simulink model "ControlSM_Tilt"  (R2013b)
settings: Solver=FixedStepDiscrete  StartTime=0.0  StopTime=10.0  FixedStep=0.001  RelTol=1e-3
undefined symbols (not defined in the file): B0, B13, B14, B3, C0, C9, DiscIntNeverNeededParam, P0, P13, P14, P16, P25, P3, Pin, Timer
libraries: MCHP_Blockset x13, simulink x1
settings Model: Creator=Residente  LastModifiedBy=Maestria01
settings OptimizationCC: InlineParams=on  InlineInvariantSignals=on  OptimizeModelRefInitCode=on  LifeSpan=1
settings HardwareCC: ProdBitPerInt=16  ProdBitPerPointer=16  ProdLargestAtomicInteger=Integer  ProdIntDivRoundTo=Zero  ProdEndianess=LittleEndian  ProdWordSize=16  ProdHWDeviceType=Generic->Custom
settings RTWCC: SystemTargetFile=MCHP_dsPIC_stf.tlc  TemplateMakefile=MCHP_dsPIC.tmf  Description=Microchip Embedded Target PIC24 dsPIC30 dsPIC33 (real-time)  ProcessScript=MCHP_dsPIC_stf_make_rtw_hook  CustomInclude=./Source  CustomSource=receive.c
settings CodeAppCC: IgnoreCustomStorageClasses=off
settings STFCustomTargetCC: TargetLibSuffix=_lib.a  IncludeMdlTerminateFcn=off  CombineOutputUpdateFcns=on  SuppressErrorStatus=on  ERTCustomFileBanners=on  SupportContinuousTime=off  MATLABClassNameForMDSCustomization=Simulink.SoftwareTarget.ERTCustomization  GRTInterface=off  SystemTargetFile=MCHP_dsPIC_stf.tlc
settings ERTTargetCC: TargetLibSuffix=_lib.a  CodeReplacementLibrary=ANSI_C  ParMdlRefBuildCompliant=off  CompOptLevelCompliant=off  ConcurrentExecutionCompliant=off  IncludeMdlTerminateFcn=off  SuppressErrorStatus=on  ERTFirstTimeCompliant=off  SupportNonInlinedSFcns=on  ModelStepFunctionPrototypeControlCompliant=off  CPPClassGenCompliant=off  InlinedParameterPlacement=NonHierarchical  ERTSrcFileBannerTemplate=MCHP_dsPIC_code_template.cgt  ERTHdrFileBannerTemplate=MCHP_dsPIC_code_template.cgt  ERTDataSrcFileTemplate=MCHP_dsPIC_code_template.cgt  ERTDataHdrFileTemplate=MCHP_dsPIC_code_template.cgt  ERTCustomFileTemplate=MCHP_main.tlc

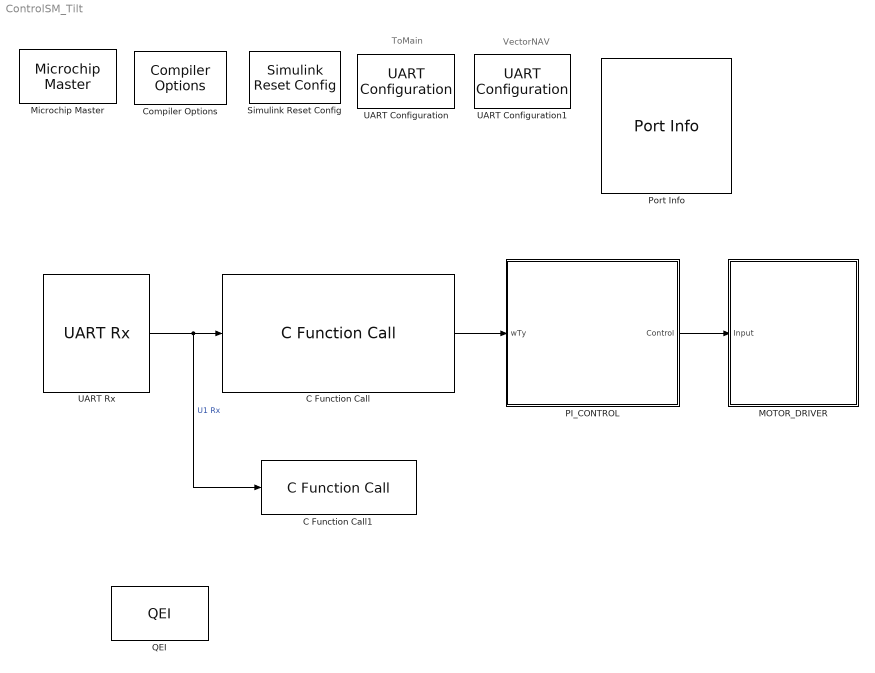
== system ControlSM_Tilt ==
  note: VectorNAV
  note: ToMain
  C Function Call : MCHP_Blockset/User Functions/C Function Call  ParseFilesChkbx=on  ListFunctions1=Custom Function  Function1=double Receive_wTy(unsigned char data[])  AddHeaderDeclaration=on  Function1Type=when block is updated (default)  Fct1BlockIn=data  FctReturnBlockOut=on  DataCollected="s.chksm={ '205028-abr-2015 10:34:56'};s.File1=reshape({ '  void  WriteUART(unsigned char data)','  void  send_wTy(unsigned char data[])','  double  Receive_wTy(unsigned char data[])','  void  Send_float(double flt)','  double  atofloat(uint8_t *buf)'},1,5);"  ORDERING=None  SampleTime=-1  MCHP_MASTERLINK=ControlSM_Tilt/Microchip Master  PinDigitalInput=[]  PinDigitalOutput=[]  PinAnalogInput=[]
  C Function Call1 : MCHP_Blockset/User Functions/C Function Call  ParseFilesChkbx=on  ListFunctions1=Custom Function  Function1=void send_wTz(unsigned char data[])  AddHeaderDeclaration=off  Function1Type=when block is updated (default)  Fct1BlockIn=data  FctReturnBlockOut=on  DataCollected="s.chksm={ '182030-abr-2015 15:25:08'};s.File1=reshape({ '  void  WriteUART(unsigned char data)','  void  send_wTz(unsigned char data[])','  double  Receive_wTz(unsigned char data[])','  void  Send_float(double flt)','  double  atofloat(uint8_t *buf)'},1,5);"  ORDERING=None  SampleTime=-1  MCHP_MASTERLINK=ControlSM_Tilt/Microchip Master  PinDigitalInput=[]  PinDigitalOutput=[]  PinAnalogInput=[]
  Compiler Options : MCHP_Blockset/System Configuration/Compiler Options  Priority=1  LATEST_CMPLR=on  COMP_LIST=Dynamic Options  COMP_LIST_TXT=xc16 - v1.24  USE_64BIT_DOUBLE=off  MCHP_MULTITHREAD_COMPILATION=off  MCHP_MASTERLINK=ControlSM_Tilt/Microchip Master  OPTIMIZATION_LEVEL=0  MCONST=in code memory  MPLAB_LINKLIB=default  MPLAB_LINKLIB1=default  UNROLL_LOOPS=off  OMIT_FRAME_POINTER=off  PROCEDURAL_ABSTRACTION=off  HEAP_SIZE=16  OMF=elf  DEBUG_INFO=off  AssemblyListing=off  ProduceHexOutput=on
  MOTOR_DRIVER : Subsystem
  Microchip Master : MCHP_Blockset/System Configuration/Microchip Master  Priority=1  PICREF=33FJ128MC804  TIMESTEP_REF="Timer  ( 0.001s )"  BUSYFLAG=Dynamic Options  BUSYFLAG_TXT=None  PWRTEN=PWRT enabled  BOREN=Disable  BODENV=2.7V  BORV=Brown-out Reset set at 2.0V  FPWRT=16ms  DSBOREN=Deep Sleep BOR enabled in Deep Sleep  DSLPBOR=Deep Sleep BOR enabled in Deep Sleep  MCLRE=RA5 input pin disabled;MCLR pin enabled  PMDL1WAY=Allow only one reconfiguration  RSTPRI=Device will obtain reset instruction from Primary flash  TEMP=Not used  SOSCSRC=Analog Mode for use with crystal  SOSCSEL=Secondary oscillator configured for high-power operation  IOL1WAY=Allow Only One Re-configuration  ALTVREF=Voltage reference input; ADC =RA9/RA10 Comparator =RA9;RA10  DISUVREG=Regulator is disabled  DSSWEN=Deep Sleep is controlled by the register bit DSEN  LPCFG=Disabled - regardless of RETEN  RTCBAT=RTC operation is continued through VBAT  VBTBOR=VBAT BOR enabled  WUTSEL=Default regulator start-up time used  POWERSAVE=off  FNOSC=Primary oscillator (XT; HS; EC)  FPR=ECIO w/ PLL 16x  FOSFPR=HS3 w/PLL 16x  FOS=Primary Oscillator  FRANGE=High Range  OSCILLATOR_SELECT=External Clock  OSCILLATOR_SELECT_spd=External Clock  QUARTZ=27e+06  QUARTZ_spd=27e+06  ACTIV_PLL=on  ACTIV_PLL_spd=on  MIPS_DESIRED=40000000  MIPS_DESIRED_spd=40000000  FPLLMUL=24x Multiplier  FPLLIDIV=8x Divider  POSCFREQ=Primary oscillator/external clock input frequency greater than 8MHz  POSCMD=EC Oscillator Mode  POSCMOD=Primary osc disabled  MIPS=40 * 1e6  FPLLODIV=32x Divider  PLLKEN=Clock switch to PLL source will wait until the PLL lock signal is valid.  FCKSM=Clock switching is enabled; Fail-Safe Clock Monitor is disabled  FCKSMEN=Sw Disabled; Mon Disabled  IESO=Start up with FRC; then switch  DSWDTPS=1:2;147;483;648 (25.7 Days)  FWDTEN=Disable  FWDTWINSZ=Window Size is 25%  FWPSA=WDT prescaler ratio of 1:128  FWPSA0=1:128  FWPSB=1:16  WDT=Disable  WDTPOST=1:32768  WDTPRE=1:128  WDTPS=1:1048576  WINDIS=Watchdog Timer in Non-Window mode  WWDTEN=Non-Window mode  DSWDTEN=DSWDT enabled  DSWDTOSC=DSWDT uses Low Power RC Oscillator (LPRC)  FPBDIV=Pb_Clk is Sys_Clk/8  FSOSCEN=Enable SOSC  LPRCSEL=High Power; High Accuracy Mode  OSCIOFCN=OSCO/CLKO/RC15 functions as CLKO (FOSC/2)  OSCIOFNC=OSC2 pin has digital I/O function  LVRCFG=Low Voltage regulator is not available  PLL_96MHZ=Enabled  PLL96MHZ=96 MHz PLL Startup is enabled automatically on start-up  PLLDIV=PLL is disabled  WDTCLK=WDT uses LPRC  WDTCMX=WDT clock source is determined by the WDTCLK Configuration bits  WDTWIN=WDT Window is 25% of WDT period  APL=Aux Flash Code protect is disabled  APLK=Aux Flash Write Protection or Code Protection is Enabled  AWRP=Aux Flash may be written  BSS=No boot program Flash segment  BWP=Protection Disabled  BWRP=Boot Segment may be written  CP=Protection Disabled  EBS=No Boot EEPROM  ESS=No Segment Data EEPROM  GCP=General Segment Code protect is disabled  GSS=User program memory is not code-protected  GSS0=No protection  GSSK=General Segment Write Protection or Code Protection is Enabled  GWRP=General Segment may be written  PWP=Disable  RBS=No Boot RAM  RSS=No Secure RAM  SSS=No Secure Segment  SWRP=Secure segment may be written  WPCFG=Disable  WPDIS=Disable  WPEND=Write Protect from WPFP to the last page of memory  WPFP=Page 127 (0x1FC00)  ICESEL=Communicate on PGEC1/PGED1  ICS=Communicate on PGEC3 and PGED3  JTAGEN=Disable  COE=Reset Into Operational Mode  RES=Not used  DEBUG=Debugger is Disabled  BACKBUG=Not used  BKBUG=Device resets into Operational mode  ALTI2C=I2C mapped to SDA1/SCL1 pins  ALTI2C1=I2C1 mapped to SDA1/SCL1 pins  ALTI2C2=I2C2 mapped to SDA2/SCL2 pins  ALTQIO=QEA1; QEB1; INDX1 are selected as inputs to QEI1  ALTSS1=SS1A is selected as the I/O pin for SPI1  CMPPOL0=Hysteresis is applied to falling edge  CMPPOL1=Hysteresis is applied to falling edge  FCANIO=Default CAN I/O  FETHIO=Default Ethernet I/O  FMIIEN=MII Enabled  FSRSSEL=SRS Priority 7  FUSBIDIO=Controlled by the USB Module  FVBUSONIO=Controlled by USB Module  HPOL=PWM module high side output pins have active-high output polarity  HYST0=45 mV Hysteresis  HYST1=45 mV Hysteresis  I2C1SEL=Use Default SCL1/SDA1 Pins For I2C1  LPOL=PWM module low side output pins have active-high output polarity  PWMPIN=PWM module pins controlled by PORT register at device Reset  RTCOSC=RTCC uses Secondary Oscillator (SOSC)  UPLLEN=USB PLL is enabled  UPLLIDIV=12x Divider  ATMOD8=Not used  ALTPMP=EPMP pins are in default location mode  I2C2SEL=I2C2 is multiplexed to SDA2/RA3 and SCL2/RA2  ALTADREF=AVREF+/AVREF- are mapped to RA9/RA10  ALTCVREF=CVREF+/CVREF- are mapped to RA9/RA10  PWMLOCK=PWM registers may be written without key sequence  MCHP_TIMER_REQUEST={Time Step}{TS}0:2:3:1:[]:40000;  MCHP_TIMER_RESULT=[1 39998.999999999985 ]  MCHP_PLLRegisters="[25    158  16385     -1]"  MCHPVAR="MCHP.id = '33FJ128MC804';MCHP.idN = [33  128  804];MCHP.idL = {'FJ','MC',''};MCHP.Arch =3;MCHP.Rx = reshape([19  21  25  -1  -1  -1  -1  -1  -1  -1  -1  20  22  26  -1  -1  -1  -1  -1  -1  -1  -1  30  23  27  -1  -1  -1  -1  -1  -1  -1  -1  31  24  36  -1  -1  -1  -1  -1  -1  -1  -1  34  33  37  -1  -1  -1  -1  -1  -1  -1  -1  -1  41  38  -1  -1  -1  -1  -1  -1  -1  -1  -1  42   2  -1  -1  -1  -1  -1  -1  -1  -1  13  43   3  -1  -1  -1  -1  -1  -1  -1  -1  32  44   4  -1  -1  -1  -1  -1  -1  -1  -1  35   1   5  -1  -1  -1  -1  -1  -1  -1  -1  12   8  -1  -1  -1  -1  -1  -1  -1  -1  -1  -1   9  -1  -1  -1  -1  -1  -1  -1  -1  -1  -1  10  -1  -1  -1  -1  -1  -1  -1  -1  -1  -1  11  -1  -1  -1  -1  -1  -1  -1  -1  -1  -1  14  -1  -1  -1  -1  -1  -1  -1  -1  -1  -1  15  -1  -1  -1  -1  -1  -1  -1  -1  -1],11,16);MCHP.RP = [16  17  18  19  20  21  22  23  24  25  26  27  28  29  30  31  32  33  34  35  36  37  38  39  40  41];MCHP.RPI = [];MCHP.PPS.reg_RPINRx = [-1  1  1 -1 -1 -1  1  1  1  1 -1 -1 -1 -1  1  1 -1 -1 -1 -1  1  1 -1 -1  1 -1  1 -1  1  1  1 -1  1  1  1 -1  1  1  1  1  1  1  1 -1  1  1  1 -1 -1 -1 -1 -1  1];MCHP.RPINR_list = {'1','INT1','INT2','INT3','INT4','6','T2CK','T3CK','T4CK','T5CK','T6CK','T7CK','T8CK','T9CK','IC1','IC2','IC3','IC4','IC5','IC6','IC7','IC8','OCFA','OCFB','FLT1','FLT2','FLT3','FLT4','QEA1','QEB1','INDX1','HOME1','QEA2','QEB2','INDX2','HOME2','U1RX','U1CTS','U2RX','U2CTS','SDI1','SCK1','SS1','44','SDI2','SCK2','SS2','48','CSDIR','CSCK','COFSIN','52','C1RX','C2RX','U3RX','U3CTS','U4RX','U4CTS','SDI3','SCK3','SS3','62','SDI4','SCK4','SS4','66','IC9','IC10','IC11','IC12','IC13','IC14','IC15','IC16','OCFC','SYNCI1','SYNCI2','DTCMP1','DTCMP2','DTCMP3','DTCMP4','DTCMP5','DTCMP6','DTCMP7','FLT5','FLT6','FLT7','88'};MCHP.RPOR_list = {'1','C1OUT','C2OUT','U1TX','U1RTS','U2TX','U2RTS','SDO1','SCK1','SS1','SDO2','SCK2','SS2','13','14','15','C1TX','17','OC1','OC2','OC3','OC4','22','23','24','25','UPDN1','UPDN2'};MCHP.PPS.map_RPnR_RPORx = [0   1   2   3   4   5   6   7   8   9  10  11  12  13  14  15  16  17  18  19  20  21  22  23  24  25];MCHP.fcy.periph = 40000000;MCHP.TimeStepFactor = [1];MCHP.fcy.MIPS = 40000000;MCHP.TimeStep_Timer = 1;MCHP.NTIMERS = 5;MCHP.PowerSave = [0];MCHP.DMA.Num = [8];MCHP.DMA.CNTmax = [65535];MCHP.QEI.QEICONx = [49151  49151     -1     -1     -1     -1];MCHP.QEI.QEItype = [2];MCHP.QEI.Port_QEI_INDX = [-1 -1];MCHP.QEI.Port_QEI_QEA = [-1 -1];MCHP.QEI.Port_QEI_QEB = [-1 -1];MCHP.QEI.Port_QEI_UPDN = [-1 -1];MCHP.ADC.ADCONx = [63471  59327  40959      7      0      0];MCHP.ADC.ADCHS_0 = [40863   1799];MCHP.ADC.ANtype = [3  0];MCHP.ADC.Flags = [1  0];MCHP.ADC.Buffer = [1 -1];MCHP.ADC.port = [0   1  16  17  18  19  32  33  34  -1  -1  -1  -1  -1  -1  -1  -1  -1  -1  -1  -1  -1  -1  -1  -1  -1  -1  -1  -1  -1  -1  -1  -1  -1  -1  -1  -1  -1  -1  -1  -1  -1  -1  -1  -1  -1  -1  -1  -1  -1  -1  -1  -1  -1  -1  -1  -1];MCHP.ADC.port_VrefP = [-1];MCHP.ADC.port_VrefM = [-1];MCHP.ADC.port_AVdd = [-1];MCHP.ADC.port_AVss = [-1];MCHP.PWM_HS.Flags = [0  0  0];MCHP.PWM.port_FLT = [-1 -1 -1 -1 -1 -1 -1 -1 -1 -1 -1 -1 -1 -1 -1 -1 -1 -1 -1 -1 -1 -1 -1 -1 -1 -1 -1 -1 -1 -1 -1 -1 -1];MCHP.PWM.PWMRef = 2;MCHP.PWM.Flag = 2;MCHP.PWM.Port_PWM_l = [31  29  27  -1  -1  -1  -1  -1  -1;39  -1  -1  -1  -1  -1  -1  -1  -1];MCHP.PWM.Port_PWM_h = [30  28  26  -1  -1  -1  -1  -1  -1;38  -1  -1  -1  -1  -1  -1  -1  -1];MCHP.IC.Port = [32767  32767      0      0      0      0  32767  32767      0      0      0      0      0      0      0      0];MCHP.IC.type = 0;MCHP.OC.Port = [32767  32767  32767  32767      0      0  32767  32767      0      0      0      0      0      0      0      0];MCHP.OC.type = 0;MCHP.CN.Port = [4  20   0   1  16  17  18  19  32  33  34  31  30  29  28  27  26  39  38  41  40  25  24  23  22  36  37  21  35   3   2  -1  -1  -1  -1  -1  -1  -1  -1  -1  -1  -1  -1  -1  -1  -1  -1  -1  -1  -1  -1  -1  -1  -1  -1  -1  -1  -1  -1  -1  -1  -1  -1  -1  -1  -1  -1  -1  -1  -1  -1  -1  -1  -1  -1  -1  -1  -1  -1  -1  -1  -1  -1  -1  -1];MCHP.CN.PullUp = [65535  32767      0      0      0      0      0      0      0      0      0];MCHP.CN.type = 0;MCHP.CN.Flag_PullDown = 1;MCHP.SPI.Refs = [1  2  0  0  0  0];MCHP.SPI.SPIxCON1 = 8191;MCHP.SPI.SPIxCON2 = 57346;MCHP.SPI.Port_SDI = [-1 -1 -1 -1 -1 -1];MCHP.SPI.Port_SDO = [-1 -1 -1 -1 -1 -1];MCHP.SPI.Port_SCK = [-1 -1 -1 -1 -1 -1];MCHP.SPI.Port_SS = [-1 -1 -1 -1 -1 -1];MCHP.I2C.Refs = [1  0  0  0  0];MCHP.I2C.I2CxCON = 65535;MCHP.I2C.NewRegName = 1;MCHP.I2C.Port_SDA = [25  -1  -1  -1  -1];MCHP.I2C.Port_SCL = [24  -1  -1  -1  -1];MCHP.I2C.Port_ASDA = [21  -1  -1  -1  -1];MCHP.I2C.Port_ASCL = [22  -1  -1  -1  -1];MCHP.I2C.Fuse_Port_SCL_SDA = [20  -1  -1  -1  -1;1 -1 -1 -1 -1];MCHP.I2C.Fuse_Port_ASCL_ASDA = [20  -1  -1  -1  -1;2 -1 -1 -1 -1];MCHP.Comp.Port_CVrefin = [-1];MCHP.Comp.Port_CVref = [34];MCHP.Comp.Port_CVref1O = [-1];MCHP.Comp.Port_CVref2O = [-1];MCHP.Comp.Port_CxOUT = [-1 -1 -1 -1 -1];MCHP.Comp.Port_OAxOUT = [-1 -1 -1 -1 -1];MCHP.Comp.Port_CxINP = [19  17  -1  -1  -1];MCHP.Comp.Port_CxINM = [-1 -1 -1 -1;-1 -1 -1 -1;-1 -1 -1 -1;-1 -1 -1 -1;-1 -1 -1 -1];MCHP.Comp.nComp = [0  0  2];MCHP.Comp.OpAmp = [0];MCHP.Comp.CVRCON = [255    0];MCHP.UART.port_Rx = [32767  32767     -1     -1     -1     -1];MCHP.UART.port_Tx = [32767  32767     -1     -1     -1     -1];MCHP.UART.port_ARx = [-1 -1];MCHP.UART.port_ATx = [-1 -1];MCHP.UART.port_RTS = [32767  32767     -1     -1     -1     -1];MCHP.UART.port_CTS = [32767  32767     -1     -1     -1     -1];MCHP.UART.reg_UxMODE = [64511  64511     -1     -1     -1     -1];MCHP.UART.reg_UxSTA = [61439  61439     -1     -1     -1     -1];"  MCHP_CRC=1216930  BTMODE=Device is in Single Boot (legacy) mode  RES1=Not used  PLLSS=PLL is fed by the Primary oscillator  RES2=Not used  ALTCMPI=C1INC is on RB13; C2INC is on RB9 and C3INC is on RA0  BOREN1=BOR Enabled [When BOREN=1]  ALTRB6=Append the RP6/ASCL1/PMPD6 functions of RB6 to RA1 pin functions  RETCFG=Retention regulator is not available  DFMCY=48 Tcy  BSS2=No Boot Segment  CWRP=Configuration Segment may be written  CSS=No Protection (other than CWRP)  AIVTDIS=Disable Alternate Vector Table  BSLIM=Not used  WDTEN=Disable  BTSWP=Not used  DBCC=Not used  CTXT1=Not Assigned  CTXT2=Not Assigned  SEQNUM=Not used  nSEQNUM=Not used  BOREN0=Enabled  DMTIVT=Not used  DMTCNT=2^31 (2147483648)  DMTEN=Dead Man Timer is Enabled and cannot be disabled by software  ON=Not used  USERID=Not used  RESERVED1=Not used  PGL1WAY=Allow only one reconfiguration  FPLLRNG=34-68 MHz Input  FPLLICLK=FRC is input to the System PLL  FPLLMULT=PLL Multiply by 128  UPLLFSEL=USB PLL input is 24 MHz  DMTINTV=Window/Interval value is 127/128 counter value  WDTSPGM=WDT stops during Flash programming  FDMTEN=Deadman Timer is disabled  TRCEN=Trace features in the CPU are enabled  BOOTISA=Boot code and Exception code is MIPS32  FECCCON=ECC and Dynamic ECC are disabled (ECCCON bits are writable)  FSLEEP=Flash is powered down when the device is in Sleep mode  DBGPER=Allow CPU access to all permission regions  EJTAGBEN=Normal EJTAG functionality  TSEQ=Not used  CSEQ=Not used
  PI_CONTROL : Subsystem
  Port Info : MCHP_Blockset/System Info/Port Info  MCHP_MASTERLINK=ControlSM_Tilt/Microchip Master
  QEI : MCHP_Blockset/QEI/QEI  QEI_REF=1  QEI_MODE=Quadrature Encoder  QEI_x2mode=off  QEI_PulseCountDir=Down  PIN_QEA=Dynamic Options  PIN_QEA_TXT=B0 / P0 / Pin[21]  PIN_QEB=Dynamic Options  PIN_QEB_TXT=B0 / P0 / Pin[21]  SWPAB=off  QEAPOL=off  QEBPOL=off  SampleTime=.001  INDXxCNT_Output=is not an output  POSxCNT_Output=is a 16 bits unsigned block output  RESET_Input=off  PIMOD_mode=Never reset position  PIMOD_modeB=Never reset position  PIMOD_reset=on next INDEX event  PIN_INDEX=Dynamic Options  PIN_INDEX_TXT=B0 / P0 / Pin[21]  IMV=QEA = 1 and QEB = 0  PIN_HOME=Dynamic Options  PIN_HOME_TXT=B0 / P0 / Pin[21]  QEIxLEC_GEC=[0 200]  QEIxIC=52  PCIIRQ=off  IDXPOL=off  HOMPOL=on  VELxCNT_Output=is a 16 bits unsigned block output  INTxHLD_Output=is not an output  MaxPeriod=1e-3  FILTREN=on  QFDIV_popup=Dynamic Options  QFDIV_popup_TXT=52.08 kHz  FILTER_CutOffFreq=100e3  PIN_CCMP=Dynamic Options  PIN_CCMP_TXT=B0 / P0 / Pin[21]  MCHP_PORT={QEI1 A}{QEA1}5:0:P0;{QEI1 B}{QEB1}5:0:P0;  MCHP_MASTERLINK=ControlSM_Tilt/Microchip Master  QEI_IntPri=5
  Simulink Reset Config : MCHP_Blockset/System Configuration/Simulink Reset Config  MCHP_MASTERLINK=0
  UART Configuration : MCHP_Blockset/BUS UART/UART Configuration  UART_REF=2  BAUD_Choice=Dynamic Options  BAUD_Choice_TXT="115200         [-0.22%]"  BAUD_Choice_IR=Dynamic Options  BAUD_Choice_IR_TXT=[]  BAUD_Custom=115200  IRDA=off  ALT_IO=on  PIN_RX=Dynamic Options  PIN_RX_TXT=B3 / P3 / Pin[24]  PIN_TX=Dynamic Options  PIN_TX_TXT=C0 / P16 / Pin[25]  FlowControl=None  PIN_CTS=Dynamic Options  PIN_CTS_TXT=B0 / P0 / Pin[21]  PIN_RTS=Dynamic Options  PIN_RTS_TXT=B0 / P0 / Pin[21]  MCHP_PORT="{UART2  Rx}{U2RX}3:0:P3;{UART2  Tx}{U2TX}3:1:P16;"  TX_IMPLEMENTATION=Simplest (4 bytes internal buffer only)  TX_INT_PRIORITY=1  TX_INT_WHEN=is empty & last char is sent  TX_CIRCULAR_SIZE=128  TX_DMA_CHANNEL="0   (Lowest Priority)"  TX_DMA_SIZE=[]  RX_IMPLEMENTATION=Simplest (4 bytes internal buffer only)  RX_INT_PRIORITY=1  RX_INT_WHEN=receive 1 character  RX_CIRCULAR_SIZE=32  InitSequence_chkbox=off  BAUD_Choice_InitSeq=Dynamic Options  BAUD_Choice_InitSeq_TXT="110         [+0.00%]"  BAUD_Choice_IR_InitSeq=Dynamic Options  BAUD_Choice_IR_InitSeq_TXT=0  BAUD_Custom_InitSeq=0  InitSequence='Hello World'  MCHP_MASTERLINK=ControlSM_Tilt/Microchip Master
  UART Configuration1 : MCHP_Blockset/BUS UART/UART Configuration  UART_REF=1  BAUD_Choice=Dynamic Options  BAUD_Choice_TXT="115200         [-0.22%]"  BAUD_Choice_IR=Dynamic Options  BAUD_Choice_IR_TXT=[]  BAUD_Custom=115200  IRDA=off  ALT_IO=on  PIN_RX=Dynamic Options  PIN_RX_TXT=B14 / P14 / Pin[14]  PIN_TX=Dynamic Options  PIN_TX_TXT=B13 / P13 / Pin[11]  FlowControl=None  PIN_CTS=Dynamic Options  PIN_CTS_TXT=B0 / P0 / Pin[21]  PIN_RTS=Dynamic Options  PIN_RTS_TXT=B0 / P0 / Pin[21]  MCHP_PORT="{UART1  Rx}{U1RX}3:0:P14;{UART1  Tx}{U1TX}3:1:P13;"  TX_IMPLEMENTATION=Circular Buffer  TX_INT_PRIORITY=1  TX_INT_WHEN=is empty & last char is sent  TX_CIRCULAR_SIZE=128  TX_DMA_CHANNEL="0   (Lowest Priority)"  TX_DMA_SIZE=[]  RX_IMPLEMENTATION=Circular Buffer  RX_INT_PRIORITY=3  RX_INT_WHEN=receive 1 character  RX_CIRCULAR_SIZE=128  InitSequence_chkbox=off  BAUD_Choice_InitSeq=Dynamic Options  BAUD_Choice_InitSeq_TXT="115200         [-0.22%]"  BAUD_Choice_IR_InitSeq=Dynamic Options  BAUD_Choice_IR_InitSeq_TXT=0  BAUD_Custom_InitSeq=0  InitSequence='$VNWRG,6,0*XX'  MCHP_MASTERLINK=ControlSM_Tilt/Microchip Master
  UART Rx : MCHP_Blockset/BUS UART/UART Rx  UART_REF=1  Flag_Out=off  Rx_Size=128  Split=Read all received char  SplitChar=*  OutputDefault_popup=Add one trailing 0  OutputDefault=-2  ORDERING=None  SampleTime=0.025  MCHP_MASTERLINK=ControlSM_Tilt/Microchip Master
  wires:
  UART Rx/1 -> C Function Call1/1, C Function Call/1  "U1 Rx"
  C Function Call/1 -> PI_CONTROL/1(wTy)
  PI_CONTROL/1(Control) -> MOTOR_DRIVER/1(Input)

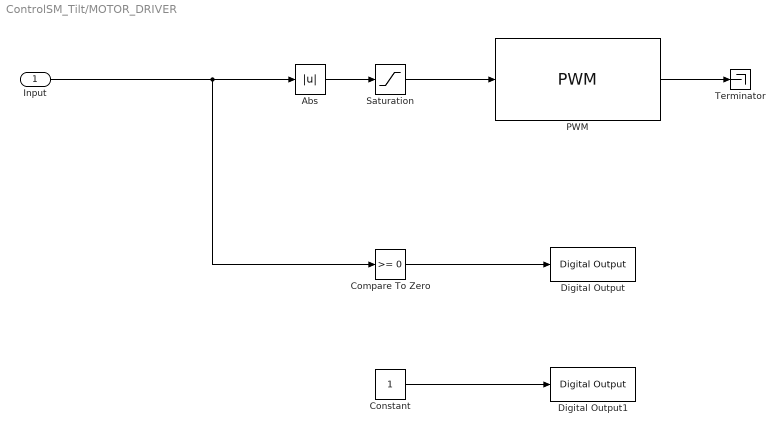
== system ControlSM_Tilt/MOTOR_DRIVER ==
  Input : Inport
  Abs : Abs  OutDataTypeStr=uint16
  Compare To Zero : simulink/Logic and Bit Operations/Compare To Zero  relop=>=  OutDataTypeStr=boolean
  Constant : Constant  OutDataTypeStr=boolean
  Digital Output : MCHP_Blockset/Digital IO/Digital Output  PORT=Dynamic Options  PORT_TXT="B   [ 0 : 15 ]"  PIN=[11]  PACK=off  SIMULTANEOUS=off  READPREVIOUS=off  ORDERING=None  SampleTime=-1  MCHP_MASTERLINK=ControlSM_Tilt/Microchip Master
  Digital Output1 : MCHP_Blockset/Digital IO/Digital Output  PORT=Dynamic Options  PORT_TXT="C   [ 0 : 9 ]"  PIN=[8]  PACK=off  SIMULTANEOUS=off  READPREVIOUS=off  ORDERING=None  SampleTime=-1  MCHP_MASTERLINK=ControlSM_Tilt/Microchip Master
  PWM : MCHP_Blockset/PWM IO/PWM  PWM_REF=1  ChannelHighLowChk=on  Channel=[]  ChannelHigh=[2]  InitialPeriod=.00005  InputPeriodeChk=off  CAM=off  IUE=on  Info="PWM1max = 3997  ;   % ==>  11.9647 bits"  MCHP_MASTERLINK=ControlSM_Tilt/Microchip Master  MCHP_PORT={PWM1 Fault A}{FLT1}5:0:P25;{PWM_H2}{PWM_H}5:1:B12;  ADC_VARTRIG={PWM Primary Special Event Trigger;6}  SampleTime=-1  DeadTimePrescaleA=0  DeadTimePrescaleB=0  DTPWM1a=Prescaler A  DTPWM1i=Prescaler B  DTPWM2a=Prescaler A  DTPWM2i=Prescaler A  DTPWM3a=Prescaler A  DTPWM3i=Prescaler A  DTPWM4a=Prescaler A  DTPWM4i=Prescaler A  PIN_FaultA=Dynamic Options  PIN_FaultA_TXT=C9 / P25 / Pin[5]  FAULTA_FLATM=Re-Enable PWM when Fault Pin is desactivated  FaultA_Output=on  FaultA_PWM1_State=No Changes (PWM)  FaultA_PWM2_State=No Changes (PWM)  FaultA_PWM3_State=No Changes (PWM)  FaultA_PWM4_State=No Changes (PWM)  PIN_FaultB=Dynamic Options  PIN_FaultB_TXT=B0 / P0 / Pin[21]  FAULTB_FLBTM=Re-Enable PWM when Fault Pin is desactivated  FaultB_Output=off  FaultB_PWM1_State=No Changes (PWM)  FaultB_PWM2_State=No Changes (PWM)  FaultB_PWM3_State=No Changes (PWM)  FaultB_PWM4_State=No Changes (PWM)  PxSECMP=.000005  PxSECMPBlkInChk=off  OVDCONChk=off
  Saturation : Saturate  UpperLimit=3997  LowerLimit=0
  Terminator : Terminator
  wires:
  Compare To Zero/1 -> Digital Output/1
  Input/1 -> Compare To Zero/1, Abs/1
  Constant/1 -> Digital Output1/1
  PWM/1 -> Terminator/1
  Saturation/1 -> PWM/1
  Abs/1 -> Saturation/1

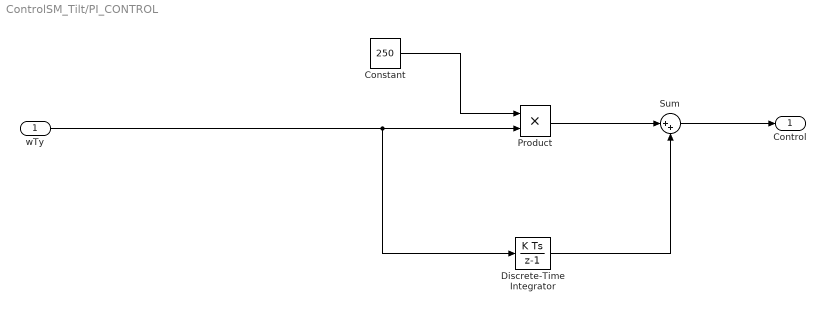
== system ControlSM_Tilt/PI_CONTROL ==
  wTy : Inport
  Constant : Constant  Value=250
  Discrete-Time Integrator : DiscreteIntegrator  gainval=750  SampleTime=-1  ICPrevOutput=DiscIntNeverNeededParam  ICPrevScaledInput=DiscIntNeverNeededParam
  Product : Product
  Sum : Sum  Inputs=|++
  Control : Outport
  wires:
  Sum/1 -> Control/1
  Product/1 -> Sum/1
  Constant/1 -> Product/1
  Discrete-Time Integrator/1 -> Sum/2
  wTy/1 -> Discrete-Time Integrator/1, Product/2
